simulink model "matlab_ros_com_formation1"  (R2017b)
settings: Solver=VariableStepAuto  StartTime=0.0  StopTime=inf  FixedStep=0.001  RelTol=1e-3  EnableMultiTasking=on
InitFcn:
  | sub_pose_time=0.1;
  | sub_vel_time=0.1;
  | pub_vel_time=0.1;
  | pub_pose_time=0.1;
  | 
  | Simulink.importExternalCTypes('uav.h');
undefined symbols (not defined in the file or in its folder): Pose, Twist
libraries: robotlib x28, simulink x1
settings Model: Creator=Administrator  LastModifiedBy=shitou
settings OptimizationCC: LifeSpan=inf
settings DebuggingCC: SFUnexpectedBacktrackingDiag=warning  SFNoUnconditionalDefaultTransitionDiag=warning  SFExecutionAtInitializationDiag=none
settings SFSimCC: SimCustomHeaderCode=#include <uav.h>
settings CodeAppCC: StateflowObjectComments=on
settings GRTTargetCC: TargetLangStandard=C89/C90 (ANSI)  GeneratePreprocessorConditionals=Disable all
settings ConfigComp: CovMetricSettings=dw  CovHtmlReporting=on  CovSaveCumulativeToWorkspaceVar=on  CovSaveSingleToWorkspaceVar=on  CovExternalEMLEnable=off

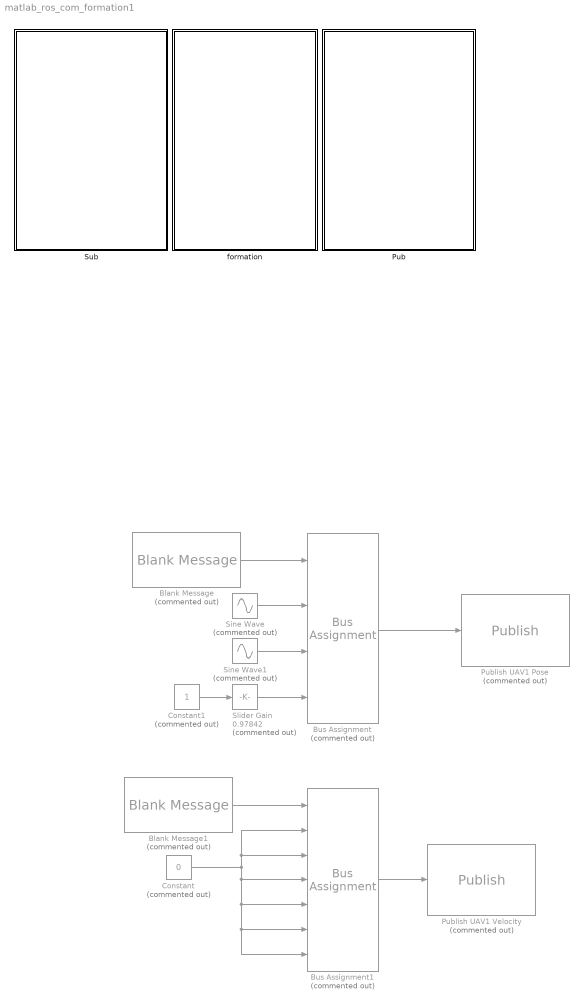
== system matlab_ros_com_formation1 ==
  Blank Message : robotlib/Blank Message  Commented=on  SourceLibraryInfo=This block requires Robotics System Toolbox  messageType=geometry_msgs/PoseStamped  SampleTime=-1
      settings: SourceProductBaseCode=RO
  Blank Message1 : robotlib/Blank Message  Commented=on  SourceLibraryInfo=This block requires Robotics System Toolbox  messageType=geometry_msgs/TwistStamped  SampleTime=inf
      settings: SourceProductBaseCode=RO
  Bus Assignment : BusAssignment  Commented=on  AssignedSignals=Pose.Position.X,Pose.Position.Y,Pose.Position.Z
  Bus Assignment1 : BusAssignment  Commented=on  AssignedSignals=Twist.Linear.X,Twist.Linear.Y,Twist.Linear.Z,Twist.Angular.X,Twist.Angular.Y,Twist.Angular.Z
  Constant : Constant  Commented=on  Value=0
  Constant1 : Constant  Commented=on
  Pub : Subsystem
  Publish UAV1 Pose : robotlib/Publish  Commented=on  SourceLibraryInfo=This block requires Robotics System Toolbox  topicSource=Specify your own  topic=uav1_matlab/mavros/local_position/pose  messageType=geometry_msgs/PoseStamped  messageQueueLength=1
      settings: SourceProductBaseCode=RO
  Publish UAV1 Velocity : robotlib/Publish  Commented=on  SourceLibraryInfo=This block requires Robotics System Toolbox  topicSource=Specify your own  topic=uav1_matlab/mavros/local_position/velocity_local  messageType=geometry_msgs/TwistStamped  messageQueueLength=1
      settings: SourceProductBaseCode=RO
  Sine Wave : Sin  Commented=on  Frequency=0.05*pi
  Sine Wave1 : Sin  Commented=on  Frequency=0.05*pi  Phase=pi/2
  Slider Gain : simulink/Math Operations/Slider Gain  Commented=on  gain=0.97842  low=0  high=2
  Sub : Subsystem
  formation : Subsystem
  wires:
  Blank Message/1 -> Bus Assignment/1
  Bus Assignment/1 -> Publish UAV1 Pose/1
  Blank Message1/1 -> Bus Assignment1/1
  Bus Assignment1/1 -> Publish UAV1 Velocity/1
  Constant1/1 -> Slider Gain/1
  Slider Gain/1 -> Bus Assignment/4
  Sine Wave/1 -> Bus Assignment/2
  Sine Wave1/1 -> Bus Assignment/3
  Constant/1 -> Bus Assignment1/7, Bus Assignment1/6, Bus Assignment1/5, Bus Assignment1/4, Bus Assignment1/3, Bus Assignment1/2

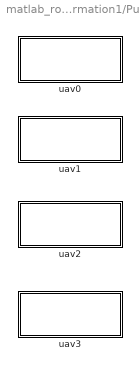
== system matlab_ros_com_formation1/Pub ==
  uav0 : Subsystem
  uav1 : Subsystem
  uav2 : Subsystem
  uav3 : Subsystem

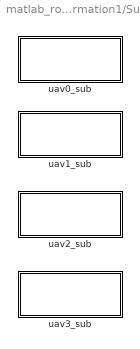
== system matlab_ros_com_formation1/Sub ==
  uav0_sub : Subsystem
  uav1_sub : Subsystem
  uav2_sub : Subsystem
  uav3_sub : Subsystem

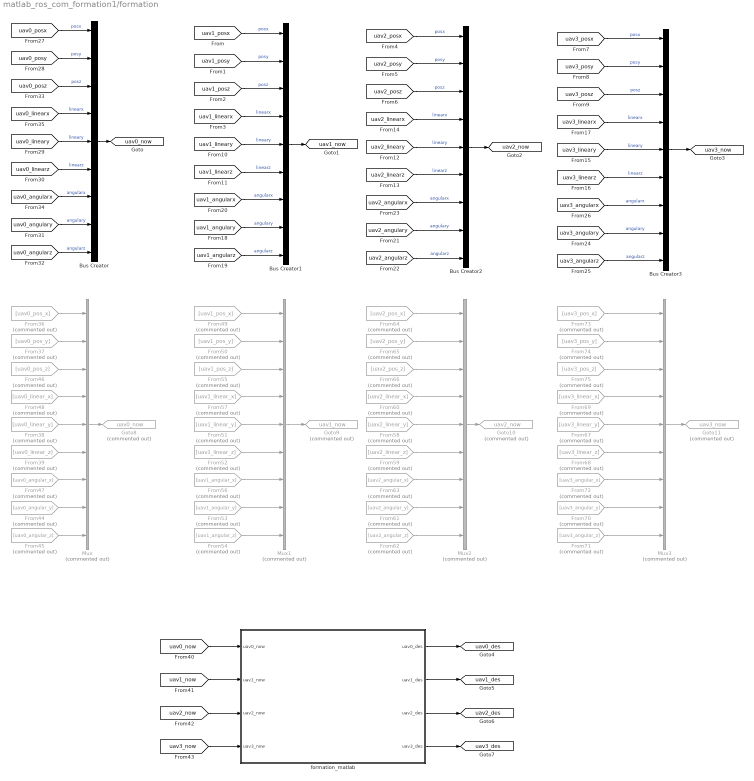
== system matlab_ros_com_formation1/formation ==
  Bus Creator{,1..3} (4 alike) : BusCreator  Inputs=9  OutDataTypeStr=Bus: uav
  From36 : From  Commented=on  GotoTag=uav0_pos_x  TagVisibility=global
  From37 : From  Commented=on  GotoTag=uav0_pos_y  TagVisibility=global
  From38 : From  Commented=on  GotoTag=uav0_linear_y  TagVisibility=global
  From39 : From  Commented=on  GotoTag=uav0_linear_z  TagVisibility=global
  From44 : From  Commented=on  GotoTag=uav0_angular_y  TagVisibility=global
  From45 : From  Commented=on  GotoTag=uav0_angular_z  TagVisibility=global
  From46 : From  Commented=on  GotoTag=uav0_pos_z  TagVisibility=global
  From47 : From  Commented=on  GotoTag=uav0_angular_x  TagVisibility=global
  From48 : From  Commented=on  GotoTag=uav0_linear_x  TagVisibility=global
  From49 : From  Commented=on  GotoTag=uav1_pos_x  TagVisibility=global
  From50 : From  Commented=on  GotoTag=uav1_pos_y  TagVisibility=global
  From51 : From  Commented=on  GotoTag=uav1_linear_y  TagVisibility=global
  From52 : From  Commented=on  GotoTag=uav1_linear_z  TagVisibility=global
  From53 : From  Commented=on  GotoTag=uav1_angular_y  TagVisibility=global
  From54 : From  Commented=on  GotoTag=uav1_angular_z  TagVisibility=global
  From55 : From  Commented=on  GotoTag=uav1_pos_z  TagVisibility=global
  From56 : From  Commented=on  GotoTag=uav1_angular_x  TagVisibility=global
  From57 : From  Commented=on  GotoTag=uav1_linear_x  TagVisibility=global
  From58 : From  Commented=on  GotoTag=uav2_linear_y  TagVisibility=global
  From59 : From  Commented=on  GotoTag=uav2_linear_z  TagVisibility=global
  From60 : From  Commented=on  GotoTag=uav2_linear_x  TagVisibility=global
  From61 : From  Commented=on  GotoTag=uav2_angular_y  TagVisibility=global
  From62 : From  Commented=on  GotoTag=uav2_angular_z  TagVisibility=global
  From63 : From  Commented=on  GotoTag=uav2_angular_x  TagVisibility=global
  From64 : From  Commented=on  GotoTag=uav2_pos_x  TagVisibility=global
  From65 : From  Commented=on  GotoTag=uav2_pos_y  TagVisibility=global
  From66 : From  Commented=on  GotoTag=uav2_pos_z  TagVisibility=global
  From67 : From  Commented=on  GotoTag=uav3_linear_y  TagVisibility=global
  From68 : From  Commented=on  GotoTag=uav3_linear_z  TagVisibility=global
  From69 : From  Commented=on  GotoTag=uav3_linear_x  TagVisibility=global
  From70 : From  Commented=on  GotoTag=uav3_angular_y  TagVisibility=global
  From71 : From  Commented=on  GotoTag=uav3_angular_z  TagVisibility=global
  From72 : From  Commented=on  GotoTag=uav3_angular_x  TagVisibility=global
  From73 : From  Commented=on  GotoTag=uav3_pos_x  TagVisibility=global
  From74 : From  Commented=on  GotoTag=uav3_pos_y  TagVisibility=global
  From75 : From  Commented=on  GotoTag=uav3_pos_z  TagVisibility=global
  Goto10 : Goto  Commented=on  GotoTag=uav2_now  TagVisibility=global
  Goto11 : Goto  Commented=on  GotoTag=uav3_now  TagVisibility=global
  Goto8 : Goto  Commented=on  GotoTag=uav0_now  TagVisibility=global
  Goto9 : Goto  Commented=on  GotoTag=uav1_now  TagVisibility=global
  Mux{,1..3} (4 alike) : Mux  Commented=on  Inputs=9
  formation_matlab : MATLAB Function  TreatAsAtomicUnit=on
  tag scope: uav0_des=global, uav0_now=global, uav1_des=global, uav1_now=global, uav2_des=global, uav2_now=global, uav3_des=global, uav3_now=global
  wires:
  [uav0_posx] -> Bus Creator/1  "posx"
  [uav0_posy] -> Bus Creator/2  "posy"
  [uav0_posz] -> Bus Creator/3  "posz"
  [uav0_linearx] -> Bus Creator/4  "linearx"
  [uav0_lineary] -> Bus Creator/5  "lineary"
  [uav0_linearz] -> Bus Creator/6  "linearz"
  [uav0_angularx] -> Bus Creator/7  "angularx"
  [uav0_angulary] -> Bus Creator/8  "angulary"
  [uav0_angularz] -> Bus Creator/9  "angularz"
  Bus Creator/1 -> [uav0_now]
  [uav1_posx] -> Bus Creator1/1  "posx"
  [uav1_posz] -> Bus Creator1/3  "posz"
  [uav1_posy] -> Bus Creator1/2  "posy"
  [uav1_linearx] -> Bus Creator1/4  "linearx"
  [uav1_lineary] -> Bus Creator1/5  "lineary"
  [uav1_linearz] -> Bus Creator1/6  "linearz"
  [uav1_angularz] -> Bus Creator1/9  "angularz"
  [uav1_angulary] -> Bus Creator1/8  "angulary"
  [uav1_angularx] -> Bus Creator1/7  "angularx"
  [uav2_posx] -> Bus Creator2/1  "posx"
  [uav2_posy] -> Bus Creator2/2  "posy"
  [uav2_posz] -> Bus Creator2/3  "posz"
  [uav2_linearx] -> Bus Creator2/4  "linearx"
  [uav2_lineary] -> Bus Creator2/5  "lineary"
  [uav2_linearz] -> Bus Creator2/6  "linearz"
  [uav2_angularx] -> Bus Creator2/7  "angularx"
  [uav2_angulary] -> Bus Creator2/8  "angulary"
  [uav2_angularz] -> Bus Creator2/9  "angularz"
  [uav3_posx] -> Bus Creator3/1  "posx"
  [uav3_angularz] -> Bus Creator3/9  "angularz"
  [uav3_angulary] -> Bus Creator3/8  "angulary"
  [uav3_angularx] -> Bus Creator3/7  "angularx"
  [uav3_linearz] -> Bus Creator3/6  "linearz"
  [uav3_lineary] -> Bus Creator3/5  "lineary"
  [uav3_linearx] -> Bus Creator3/4  "linearx"
  [uav3_posz] -> Bus Creator3/3  "posz"
  [uav3_posy] -> Bus Creator3/2  "posy"
  Bus Creator1/1 -> [uav1_now]
  Bus Creator2/1 -> [uav2_now]
  Bus Creator3/1 -> [uav3_now]
  [uav0_now] -> formation_matlab/1(uav0_now)
  [uav1_now] -> formation_matlab/2(uav1_now)
  [uav2_now] -> formation_matlab/3(uav2_now)
  [uav3_now] -> formation_matlab/4(uav3_now)
  formation_matlab/2(uav1_des) -> [uav1_des]
  formation_matlab/3(uav2_des) -> [uav2_des]
  formation_matlab/4(uav3_des) -> [uav3_des]
  From44/1 -> Mux/8
  From47/1 -> Mux/7
  From45/1 -> Mux/9
  From39/1 -> Mux/6
  From38/1 -> Mux/5
  From46/1 -> Mux/3
  From37/1 -> Mux/2
  From36/1 -> Mux/1
  From48/1 -> Mux/4
  Mux/1 -> Goto8/1
  From57/1 -> Mux1/4
  From54/1 -> Mux1/9
  From56/1 -> Mux1/7
  From49/1 -> Mux1/1
  From50/1 -> Mux1/2
  From53/1 -> Mux1/8
  From52/1 -> Mux1/6
  From55/1 -> Mux1/3
  From51/1 -> Mux1/5
  From60/1 -> Mux2/4
  From64/1 -> Mux2/1
  From63/1 -> Mux2/7
  From65/1 -> Mux2/2
  From61/1 -> Mux2/8
  From66/1 -> Mux2/3
  From58/1 -> Mux2/5
  From59/1 -> Mux2/6
  From62/1 -> Mux2/9
  From68/1 -> Mux3/6
  From69/1 -> Mux3/4
  From75/1 -> Mux3/3
  From73/1 -> Mux3/1
  From74/1 -> Mux3/2
  From71/1 -> Mux3/9
  From67/1 -> Mux3/5
  From70/1 -> Mux3/8
  From72/1 -> Mux3/7
  Mux1/1 -> Goto9/1
  Mux2/1 -> Goto10/1
  Mux3/1 -> Goto11/1
  formation_matlab/1(uav0_des) -> [uav0_des]

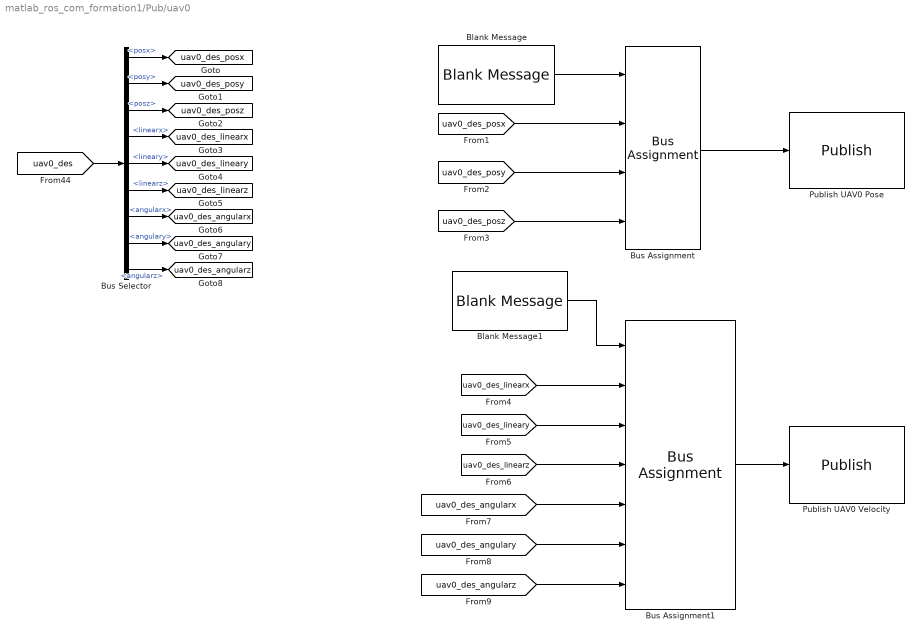
== system matlab_ros_com_formation1/Pub/uav0 ==
  Blank Message : robotlib/Blank Message  SourceLibraryInfo=This block requires Robotics System Toolbox  messageType=geometry_msgs/PoseStamped  SampleTime=pub_pose_time
      settings: SourceProductBaseCode=RO
  Blank Message1 : robotlib/Blank Message  SourceLibraryInfo=This block requires Robotics System Toolbox  messageType=geometry_msgs/TwistStamped  SampleTime=-1
      settings: SourceProductBaseCode=RO
  Bus Assignment : BusAssignment  AssignedSignals=Pose.Position.X,Pose.Position.Y,Pose.Position.Z
  Bus Assignment1 : BusAssignment  AssignedSignals=Twist.Linear.X,Twist.Linear.Y,Twist.Linear.Z,Twist.Angular.X,Twist.Angular.Y,Twist.Angular.Z
  Bus Selector : BusSelector  OutputSignals=posx,posy,posz,linearx,lineary,linearz,angularx,angulary,angularz
  Publish UAV0 Pose : robotlib/Publish  SourceLibraryInfo=This block requires Robotics System Toolbox  topicSource=Specify your own  topic=uav0_matlab/mavros/local_position/pose  messageType=geometry_msgs/PoseStamped  messageQueueLength=1
      settings: SourceProductBaseCode=RO
  Publish UAV0 Velocity : robotlib/Publish  SourceLibraryInfo=This block requires Robotics System Toolbox  topicSource=Specify your own  topic=uav0_matlab/mavros/local_position/velocity_local  messageType=geometry_msgs/TwistStamped  messageQueueLength=1
      settings: SourceProductBaseCode=RO
  tag scope: uav0_des_angularx=global, uav0_des_angulary=global, uav0_des_angularz=global, uav0_des_linearx=global, uav0_des_lineary=global, uav0_des_linearz=global, uav0_des_posx=global, uav0_des_posy=global, uav0_des_posz=global
  wires:
  Blank Message/1 -> Bus Assignment/1
  Bus Assignment/1 -> Publish UAV0 Pose/1
  Blank Message1/1 -> Bus Assignment1/1
  Bus Assignment1/1 -> Publish UAV0 Velocity/1
  [uav0_des] -> Bus Selector/1
  Bus Selector/1 -> [uav0_des_posx]  "<posx>"
  Bus Selector/3 -> [uav0_des_posz]  "<posz>"
  Bus Selector/2 -> [uav0_des_posy]  "<posy>"
  Bus Selector/4 -> [uav0_des_linearx]  "<linearx>"
  Bus Selector/5 -> [uav0_des_lineary]  "<lineary>"
  Bus Selector/6 -> [uav0_des_linearz]  "<linearz>"
  Bus Selector/7 -> [uav0_des_angularx]  "<angularx>"
  Bus Selector/8 -> [uav0_des_angulary]  "<angulary>"
  Bus Selector/9 -> [uav0_des_angularz]  "<angularz>"
  [uav0_des_posx] -> Bus Assignment/2
  [uav0_des_posy] -> Bus Assignment/3
  [uav0_des_posz] -> Bus Assignment/4
  [uav0_des_linearx] -> Bus Assignment1/2
  [uav0_des_linearz] -> Bus Assignment1/4
  [uav0_des_lineary] -> Bus Assignment1/3
  [uav0_des_angularx] -> Bus Assignment1/5
  [uav0_des_angulary] -> Bus Assignment1/6
  [uav0_des_angularz] -> Bus Assignment1/7

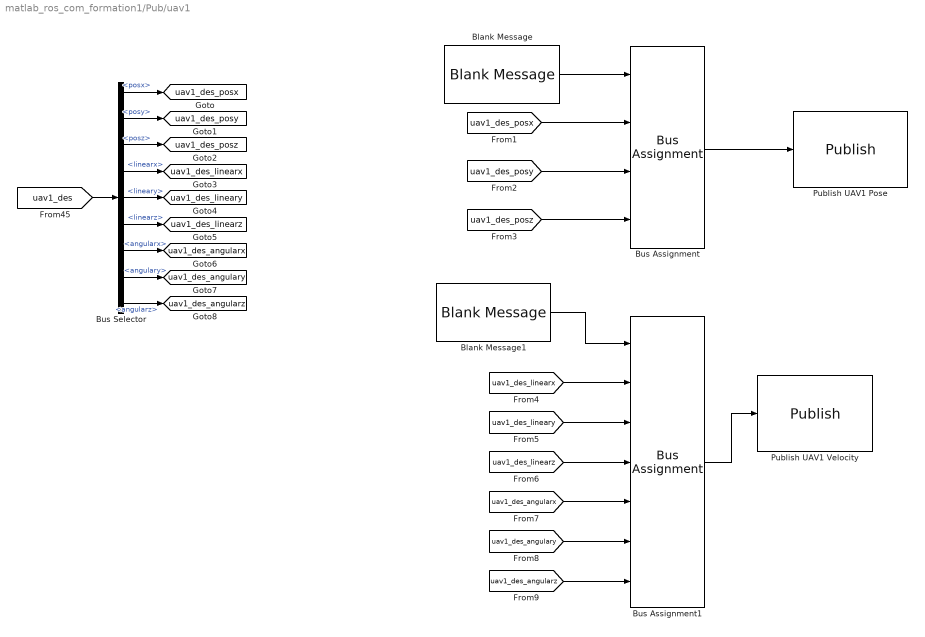
== system matlab_ros_com_formation1/Pub/uav1 ==
  Blank Message : robotlib/Blank Message  SourceLibraryInfo=This block requires Robotics System Toolbox  messageType=geometry_msgs/PoseStamped  SampleTime=pub_pose_time
      settings: SourceProductBaseCode=RO
  Blank Message1 : robotlib/Blank Message  SourceLibraryInfo=This block requires Robotics System Toolbox  messageType=geometry_msgs/TwistStamped  SampleTime=-1
      settings: SourceProductBaseCode=RO
  Bus Assignment : BusAssignment  AssignedSignals=Pose.Position.X,Pose.Position.Y,Pose.Position.Z
  Bus Assignment1 : BusAssignment  AssignedSignals=Twist.Linear.X,Twist.Linear.Y,Twist.Linear.Z,Twist.Angular.X,Twist.Angular.Y,Twist.Angular.Z
  Bus Selector : BusSelector  OutputSignals=posx,posy,posz,linearx,lineary,linearz,angularx,angulary,angularz
  Publish UAV1 Pose : robotlib/Publish  SourceLibraryInfo=This block requires Robotics System Toolbox  topicSource=Specify your own  topic=uav1_matlab/mavros/local_position/pose  messageType=geometry_msgs/PoseStamped  messageQueueLength=1
      settings: SourceProductBaseCode=RO
  Publish UAV1 Velocity : robotlib/Publish  SourceLibraryInfo=This block requires Robotics System Toolbox  topicSource=Specify your own  topic=uav1_matlab/mavros/local_position/velocity_local  messageType=geometry_msgs/TwistStamped  messageQueueLength=1
      settings: SourceProductBaseCode=RO
  tag scope: uav1_des_angularx=global, uav1_des_angulary=global, uav1_des_angularz=global, uav1_des_linearx=global, uav1_des_lineary=global, uav1_des_linearz=global, uav1_des_posx=global, uav1_des_posy=global, uav1_des_posz=global
  wires:
  Blank Message/1 -> Bus Assignment/1
  Bus Assignment/1 -> Publish UAV1 Pose/1
  Blank Message1/1 -> Bus Assignment1/1
  Bus Assignment1/1 -> Publish UAV1 Velocity/1
  [uav1_des_posz] -> Bus Assignment/4
  [uav1_des_posx] -> Bus Assignment/2
  [uav1_des_posy] -> Bus Assignment/3
  Bus Selector/2 -> [uav1_des_posy]  "<posy>"
  Bus Selector/8 -> [uav1_des_angulary]  "<angulary>"
  Bus Selector/9 -> [uav1_des_angularz]  "<angularz>"
  Bus Selector/6 -> [uav1_des_linearz]  "<linearz>"
  Bus Selector/5 -> [uav1_des_lineary]  "<lineary>"
  Bus Selector/7 -> [uav1_des_angularx]  "<angularx>"
  Bus Selector/4 -> [uav1_des_linearx]  "<linearx>"
  Bus Selector/3 -> [uav1_des_posz]  "<posz>"
  Bus Selector/1 -> [uav1_des_posx]  "<posx>"
  [uav1_des] -> Bus Selector/1
  [uav1_des_linearx] -> Bus Assignment1/2
  [uav1_des_lineary] -> Bus Assignment1/3
  [uav1_des_linearz] -> Bus Assignment1/4
  [uav1_des_angularx] -> Bus Assignment1/5
  [uav1_des_angulary] -> Bus Assignment1/6
  [uav1_des_angularz] -> Bus Assignment1/7

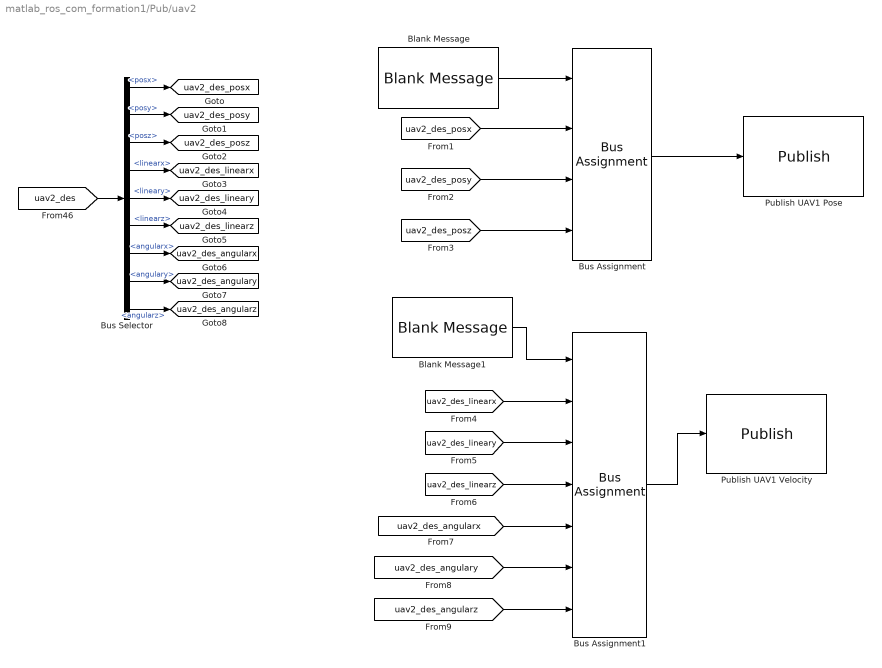
== system matlab_ros_com_formation1/Pub/uav2 ==
  Blank Message : robotlib/Blank Message  SourceLibraryInfo=This block requires Robotics System Toolbox  messageType=geometry_msgs/PoseStamped  SampleTime=pub_pose_time
      settings: SourceProductBaseCode=RO
  Blank Message1 : robotlib/Blank Message  SourceLibraryInfo=This block requires Robotics System Toolbox  messageType=geometry_msgs/TwistStamped  SampleTime=pub_vel_time
      settings: SourceProductBaseCode=RO
  Bus Assignment : BusAssignment  AssignedSignals=Pose.Position.X,Pose.Position.Y,Pose.Position.Z
  Bus Assignment1 : BusAssignment  AssignedSignals=Twist.Linear.X,Twist.Linear.Y,Twist.Linear.Z,Twist.Angular.X,Twist.Angular.Y,Twist.Angular.Z
  Bus Selector : BusSelector  OutputSignals=posx,posy,posz,linearx,lineary,linearz,angularx,angulary,angularz
  Publish UAV1 Pose : robotlib/Publish  SourceLibraryInfo=This block requires Robotics System Toolbox  topicSource=Specify your own  topic=uav2_matlab/mavros/local_position/pose  messageType=geometry_msgs/PoseStamped  messageQueueLength=1
      settings: SourceProductBaseCode=RO
  Publish UAV1 Velocity : robotlib/Publish  SourceLibraryInfo=This block requires Robotics System Toolbox  topicSource=Specify your own  topic=uav2_matlab/mavros/local_position/velocity_local  messageType=geometry_msgs/TwistStamped  messageQueueLength=1
      settings: SourceProductBaseCode=RO
  tag scope: uav2_des_angularx=global, uav2_des_angulary=global, uav2_des_angularz=global, uav2_des_linearx=global, uav2_des_lineary=global, uav2_des_linearz=global, uav2_des_posx=global, uav2_des_posy=global, uav2_des_posz=global
  wires:
  Blank Message/1 -> Bus Assignment/1
  Bus Assignment/1 -> Publish UAV1 Pose/1
  Blank Message1/1 -> Bus Assignment1/1
  Bus Assignment1/1 -> Publish UAV1 Velocity/1
  [uav2_des_linearx] -> Bus Assignment1/2
  [uav2_des_lineary] -> Bus Assignment1/3
  [uav2_des_linearz] -> Bus Assignment1/4
  [uav2_des_angularx] -> Bus Assignment1/5
  [uav2_des_angulary] -> Bus Assignment1/6
  [uav2_des_angularz] -> Bus Assignment1/7
  [uav2_des_posx] -> Bus Assignment/2
  [uav2_des_posy] -> Bus Assignment/3
  [uav2_des_posz] -> Bus Assignment/4
  Bus Selector/1 -> [uav2_des_posx]  "<posx>"
  Bus Selector/3 -> [uav2_des_posz]  "<posz>"
  Bus Selector/4 -> [uav2_des_linearx]  "<linearx>"
  Bus Selector/6 -> [uav2_des_linearz]  "<linearz>"
  Bus Selector/5 -> [uav2_des_lineary]  "<lineary>"
  Bus Selector/8 -> [uav2_des_angulary]  "<angulary>"
  Bus Selector/2 -> [uav2_des_posy]  "<posy>"
  Bus Selector/9 -> [uav2_des_angularz]  "<angularz>"
  Bus Selector/7 -> [uav2_des_angularx]  "<angularx>"
  [uav2_des] -> Bus Selector/1

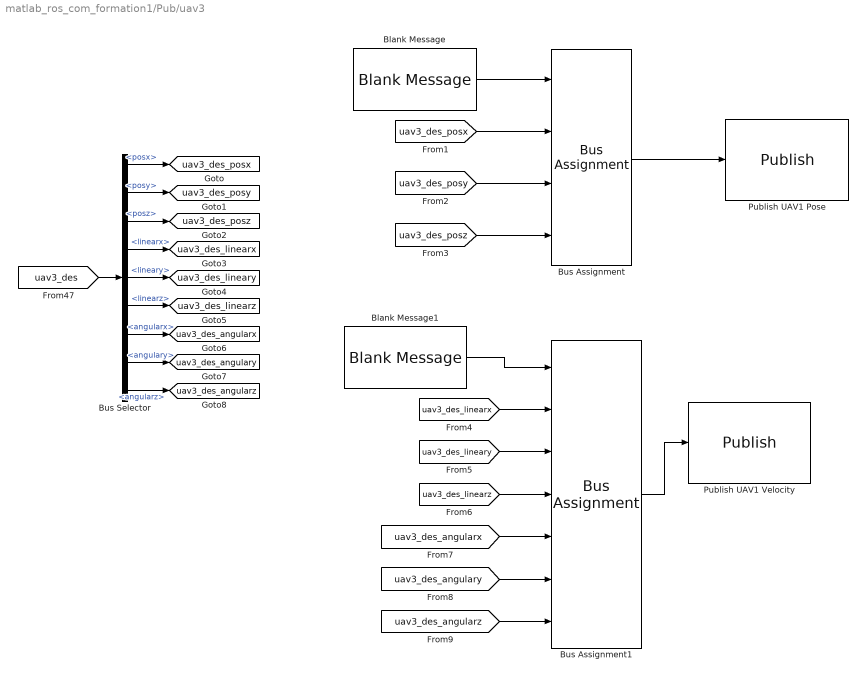
== system matlab_ros_com_formation1/Pub/uav3 ==
  Blank Message : robotlib/Blank Message  SourceLibraryInfo=This block requires Robotics System Toolbox  messageType=geometry_msgs/PoseStamped  SampleTime=pub_pose_time
      settings: SourceProductBaseCode=RO
  Blank Message1 : robotlib/Blank Message  SourceLibraryInfo=This block requires Robotics System Toolbox  messageType=geometry_msgs/TwistStamped  SampleTime=pub_vel_time
      settings: SourceProductBaseCode=RO
  Bus Assignment : BusAssignment  AssignedSignals=Pose.Position.X,Pose.Position.Y,Pose.Position.Z
  Bus Assignment1 : BusAssignment  AssignedSignals=Twist.Linear.X,Twist.Linear.Y,Twist.Linear.Z,Twist.Angular.X,Twist.Angular.Y,Twist.Angular.Z
  Bus Selector : BusSelector  OutputSignals=posx,posy,posz,linearx,lineary,linearz,angularx,angulary,angularz
  Publish UAV1 Pose : robotlib/Publish  SourceLibraryInfo=This block requires Robotics System Toolbox  topicSource=Specify your own  topic=uav3_matlab/mavros/local_position/pose  messageType=geometry_msgs/PoseStamped  messageQueueLength=1
      settings: SourceProductBaseCode=RO
  Publish UAV1 Velocity : robotlib/Publish  SourceLibraryInfo=This block requires Robotics System Toolbox  topicSource=Specify your own  topic=uav3_matlab/mavros/local_position/velocity_local  messageType=geometry_msgs/TwistStamped  messageQueueLength=1
      settings: SourceProductBaseCode=RO
  tag scope: uav3_des_angularx=global, uav3_des_angulary=global, uav3_des_angularz=global, uav3_des_linearx=global, uav3_des_lineary=global, uav3_des_linearz=global, uav3_des_posx=global, uav3_des_posy=global, uav3_des_posz=global
  wires:
  Blank Message/1 -> Bus Assignment/1
  Bus Assignment/1 -> Publish UAV1 Pose/1
  Blank Message1/1 -> Bus Assignment1/1
  Bus Assignment1/1 -> Publish UAV1 Velocity/1
  [uav3_des_posx] -> Bus Assignment/2
  [uav3_des_posy] -> Bus Assignment/3
  [uav3_des_posz] -> Bus Assignment/4
  [uav3_des_linearx] -> Bus Assignment1/2
  [uav3_des_lineary] -> Bus Assignment1/3
  [uav3_des_linearz] -> Bus Assignment1/4
  [uav3_des_angularx] -> Bus Assignment1/5
  [uav3_des_angulary] -> Bus Assignment1/6
  [uav3_des_angularz] -> Bus Assignment1/7
  Bus Selector/1 -> [uav3_des_posx]  "<posx>"
  Bus Selector/3 -> [uav3_des_posz]  "<posz>"
  Bus Selector/4 -> [uav3_des_linearx]  "<linearx>"
  Bus Selector/6 -> [uav3_des_linearz]  "<linearz>"
  Bus Selector/5 -> [uav3_des_lineary]  "<lineary>"
  Bus Selector/8 -> [uav3_des_angulary]  "<angulary>"
  Bus Selector/2 -> [uav3_des_posy]  "<posy>"
  Bus Selector/9 -> [uav3_des_angularz]  "<angularz>"
  Bus Selector/7 -> [uav3_des_angularx]  "<angularx>"
  [uav3_des] -> Bus Selector/1

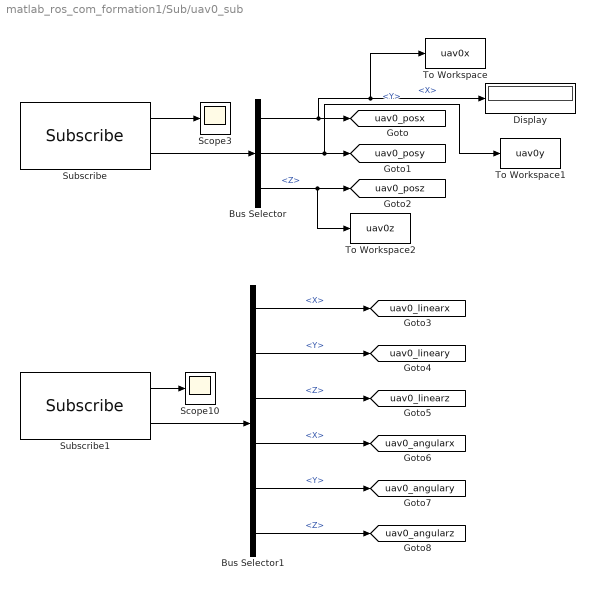
== system matlab_ros_com_formation1/Sub/uav0_sub ==
  Bus Selector : BusSelector  OutputSignals=Pose.Position.X,Pose.Position.Y,Pose.Position.Z
  Bus Selector1 : BusSelector  OutputSignals=Twist.Linear.X,Twist.Linear.Y,Twist.Linear.Z,Twist.Angular.X,Twist.Angular.Y,Twist.Angular.Z
  Display : Display
  Scope10 : Scope
  Scope3 : Scope
  Subscribe : robotlib/Subscribe  SourceLibraryInfo=This block requires Robotics System Toolbox  topicSource=Select from ROS network  topic=/uav0/mavros/local_position/pose  messageType=geometry_msgs/PoseStamped  sampleTime=sub_pose_time  messageQueueLength=1
      settings: SourceProductBaseCode=RO
  Subscribe1 : robotlib/Subscribe  SourceLibraryInfo=This block requires Robotics System Toolbox  topicSource=Select from ROS network  topic=/uav0/mavros/local_position/velocity_local  messageType=geometry_msgs/TwistStamped  sampleTime=sub_vel_time  messageQueueLength=1
      settings: SourceProductBaseCode=RO
  To Workspace : ToWorkspace  VariableName=uav0x  SaveFormat=Structure With Time  SampleTime=-1
  To Workspace1 : ToWorkspace  VariableName=uav0y  SaveFormat=Structure With Time  SampleTime=-1
  To Workspace2 : ToWorkspace  VariableName=uav0z  SaveFormat=Structure With Time  SampleTime=-1
  tag scope: uav0_angularx=global, uav0_angulary=global, uav0_angularz=global, uav0_linearx=global, uav0_lineary=global, uav0_linearz=global, uav0_posx=global, uav0_posy=global, uav0_posz=global
  wires:
  Subscribe/1 -> Scope3/1
  Subscribe/2 -> Bus Selector/1
  Bus Selector/1 -> To Workspace/1, Display/1, [uav0_posx]  "<X>"
  Bus Selector/2 -> To Workspace1/1, [uav0_posy]  "<Y>"
  Bus Selector/3 -> To Workspace2/1, [uav0_posz]  "<Z>"
  Subscribe1/2 -> Bus Selector1/1
  Subscribe1/1 -> Scope10/1
  Bus Selector1/1 -> [uav0_linearx]  "<X>"
  Bus Selector1/2 -> [uav0_lineary]  "<Y>"
  Bus Selector1/3 -> [uav0_linearz]  "<Z>"
  Bus Selector1/4 -> [uav0_angularx]  "<X>"
  Bus Selector1/5 -> [uav0_angulary]  "<Y>"
  Bus Selector1/6 -> [uav0_angularz]  "<Z>"

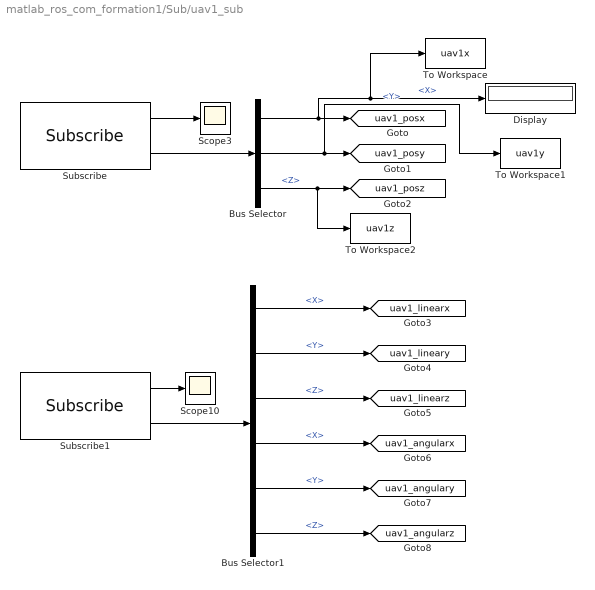
== system matlab_ros_com_formation1/Sub/uav1_sub ==
  Bus Selector : BusSelector  OutputSignals=Pose.Position.X,Pose.Position.Y,Pose.Position.Z
  Bus Selector1 : BusSelector  OutputSignals=Twist.Linear.X,Twist.Linear.Y,Twist.Linear.Z,Twist.Angular.X,Twist.Angular.Y,Twist.Angular.Z
  Display : Display
  Scope10 : Scope
  Scope3 : Scope
  Subscribe : robotlib/Subscribe  SourceLibraryInfo=This block requires Robotics System Toolbox  topicSource=Select from ROS network  topic=/uav1/mavros/local_position/pose  messageType=geometry_msgs/PoseStamped  sampleTime=sub_pose_time  messageQueueLength=1
      settings: SourceProductBaseCode=RO
  Subscribe1 : robotlib/Subscribe  SourceLibraryInfo=This block requires Robotics System Toolbox  topicSource=Select from ROS network  topic=/uav1/mavros/local_position/velocity_local  messageType=geometry_msgs/TwistStamped  sampleTime=sub_vel_time  messageQueueLength=1
      settings: SourceProductBaseCode=RO
  To Workspace : ToWorkspace  VariableName=uav1x  SaveFormat=Structure With Time  SampleTime=-1
  To Workspace1 : ToWorkspace  VariableName=uav1y  SaveFormat=Structure With Time  SampleTime=-1
  To Workspace2 : ToWorkspace  VariableName=uav1z  SaveFormat=Structure With Time  SampleTime=-1
  tag scope: uav1_angularx=global, uav1_angulary=global, uav1_angularz=global, uav1_linearx=global, uav1_lineary=global, uav1_linearz=global, uav1_posx=global, uav1_posy=global, uav1_posz=global
  wires:
  Subscribe/1 -> Scope3/1
  Subscribe/2 -> Bus Selector/1
  Bus Selector/1 -> To Workspace/1, Display/1, [uav1_posx]  "<X>"
  Bus Selector/2 -> To Workspace1/1, [uav1_posy]  "<Y>"
  Bus Selector/3 -> To Workspace2/1, [uav1_posz]  "<Z>"
  Subscribe1/2 -> Bus Selector1/1
  Subscribe1/1 -> Scope10/1
  Bus Selector1/1 -> [uav1_linearx]  "<X>"
  Bus Selector1/2 -> [uav1_lineary]  "<Y>"
  Bus Selector1/3 -> [uav1_linearz]  "<Z>"
  Bus Selector1/4 -> [uav1_angularx]  "<X>"
  Bus Selector1/5 -> [uav1_angulary]  "<Y>"
  Bus Selector1/6 -> [uav1_angularz]  "<Z>"

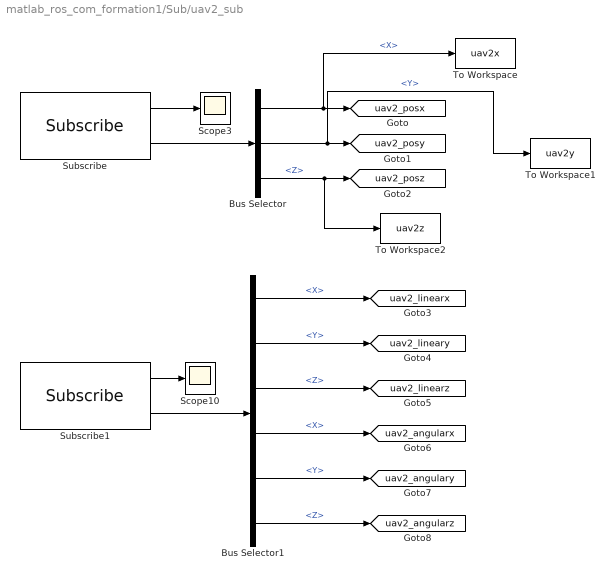
== system matlab_ros_com_formation1/Sub/uav2_sub ==
  Bus Selector : BusSelector  OutputSignals=Pose.Position.X,Pose.Position.Y,Pose.Position.Z
  Bus Selector1 : BusSelector  OutputSignals=Twist.Linear.X,Twist.Linear.Y,Twist.Linear.Z,Twist.Angular.X,Twist.Angular.Y,Twist.Angular.Z
  Scope10 : Scope
  Scope3 : Scope
  Subscribe : robotlib/Subscribe  SourceLibraryInfo=This block requires Robotics System Toolbox  topicSource=Select from ROS network  topic=/uav2/mavros/local_position/pose  messageType=geometry_msgs/PoseStamped  sampleTime=sub_pose_time  messageQueueLength=1
      settings: SourceProductBaseCode=RO
  Subscribe1 : robotlib/Subscribe  SourceLibraryInfo=This block requires Robotics System Toolbox  topicSource=Select from ROS network  topic=/uav2/mavros/local_position/velocity_local  messageType=geometry_msgs/TwistStamped  sampleTime=sub_vel_time  messageQueueLength=1
      settings: SourceProductBaseCode=RO
  To Workspace : ToWorkspace  VariableName=uav2x  SaveFormat=Structure With Time  SampleTime=-1
  To Workspace1 : ToWorkspace  VariableName=uav2y  SaveFormat=Structure With Time  SampleTime=-1
  To Workspace2 : ToWorkspace  VariableName=uav2z  SaveFormat=Structure With Time  SampleTime=-1
  tag scope: uav2_angularx=global, uav2_angulary=global, uav2_angularz=global, uav2_linearx=global, uav2_lineary=global, uav2_linearz=global, uav2_posx=global, uav2_posy=global, uav2_posz=global
  wires:
  Subscribe/1 -> Scope3/1
  Subscribe/2 -> Bus Selector/1
  Bus Selector/1 -> To Workspace/1, [uav2_posx]  "<X>"
  Bus Selector/2 -> To Workspace1/1, [uav2_posy]  "<Y>"
  Bus Selector/3 -> To Workspace2/1, [uav2_posz]  "<Z>"
  Subscribe1/2 -> Bus Selector1/1
  Subscribe1/1 -> Scope10/1
  Bus Selector1/1 -> [uav2_linearx]  "<X>"
  Bus Selector1/2 -> [uav2_lineary]  "<Y>"
  Bus Selector1/3 -> [uav2_linearz]  "<Z>"
  Bus Selector1/4 -> [uav2_angularx]  "<X>"
  Bus Selector1/5 -> [uav2_angulary]  "<Y>"
  Bus Selector1/6 -> [uav2_angularz]  "<Z>"

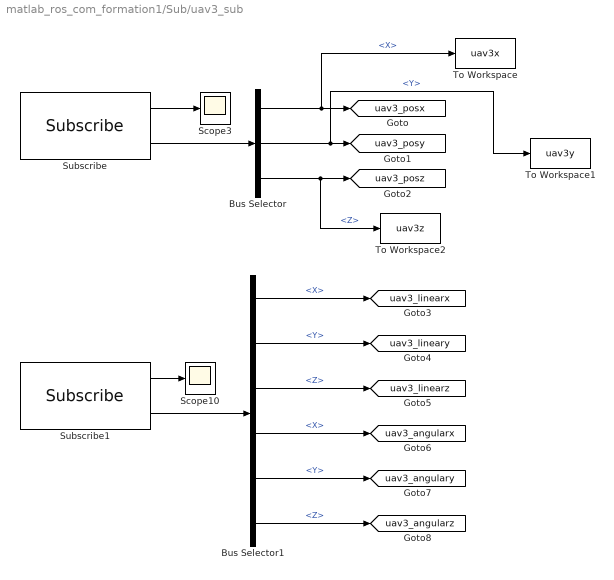
== system matlab_ros_com_formation1/Sub/uav3_sub ==
  Bus Selector : BusSelector  OutputSignals=Pose.Position.X,Pose.Position.Y,Pose.Position.Z
  Bus Selector1 : BusSelector  OutputSignals=Twist.Linear.X,Twist.Linear.Y,Twist.Linear.Z,Twist.Angular.X,Twist.Angular.Y,Twist.Angular.Z
  Scope10 : Scope
  Scope3 : Scope
  Subscribe : robotlib/Subscribe  SourceLibraryInfo=This block requires Robotics System Toolbox  topicSource=Select from ROS network  topic=/uav3/mavros/local_position/pose  messageType=geometry_msgs/PoseStamped  sampleTime=sub_pose_time  messageQueueLength=1
      settings: SourceProductBaseCode=RO
  Subscribe1 : robotlib/Subscribe  SourceLibraryInfo=This block requires Robotics System Toolbox  topicSource=Select from ROS network  topic=/uav3/mavros/local_position/velocity_local  messageType=geometry_msgs/TwistStamped  sampleTime=sub_vel_time  messageQueueLength=1
      settings: SourceProductBaseCode=RO
  To Workspace : ToWorkspace  VariableName=uav3x  SaveFormat=Structure With Time  SampleTime=-1
  To Workspace1 : ToWorkspace  VariableName=uav3y  SaveFormat=Structure With Time  SampleTime=-1
  To Workspace2 : ToWorkspace  VariableName=uav3z  SaveFormat=Structure With Time  SampleTime=-1
  tag scope: uav3_angularx=global, uav3_angulary=global, uav3_angularz=global, uav3_linearx=global, uav3_lineary=global, uav3_linearz=global, uav3_posx=global, uav3_posy=global, uav3_posz=global
  wires:
  Subscribe/1 -> Scope3/1
  Subscribe/2 -> Bus Selector/1
  Bus Selector/1 -> To Workspace/1, [uav3_posx]  "<X>"
  Bus Selector/2 -> To Workspace1/1, [uav3_posy]  "<Y>"
  Bus Selector/3 -> To Workspace2/1, [uav3_posz]  "<Z>"
  Subscribe1/2 -> Bus Selector1/1
  Subscribe1/1 -> Scope10/1
  Bus Selector1/1 -> [uav3_linearx]  "<X>"
  Bus Selector1/2 -> [uav3_lineary]  "<Y>"
  Bus Selector1/3 -> [uav3_linearz]  "<Z>"
  Bus Selector1/4 -> [uav3_angularx]  "<X>"
  Bus Selector1/5 -> [uav3_angulary]  "<Y>"
  Bus Selector1/6 -> [uav3_angularz]  "<Z>"

== matlab function matlab_ros_com_formation1/formation/formation_matlab ==
  data: uav0_now input Bus: uav; uav0_des output Bus: uav; uav1_now input Bus: uav; uav2_now input Bus: uav; uav3_now input Bus: uav; uav1_des output Bus: uav; uav2_des output Bus: uav; uav3_des output Bus: uav
function [uav0_des,uav1_des,uav2_des,uav3_des ] = formation_matlab(uav0_now,uav1_now,uav2_now,uav3_now)

% formation.Ppos_now=[uav0.now,uav1.now,uav2.now,uav3.now];
%%%%%%虚拟领导者位置
leader.posx=0;
leader.posy=0;
leader.posz=0;
T_SIZE=2.0;
k_aij=0.1;
% k_p=0.95;
k_p=1.95;


relative_pos_to_leader0.x = -T_SIZE;
relative_pos_to_leader0.y =  T_SIZE;
relative_pos_to_leader0.z = 0.0;

relative_pos_to_leader1.x =   T_SIZE;
relative_pos_to_leader1.y =   T_SIZE;
relative_pos_to_leader1.z = 0.0;
    
relative_pos_to_leader2.x =   T_SIZE;
relative_pos_to_leader2.y = - T_SIZE;
relative_pos_to_leader2.z = 0.0;
   
relative_pos_to_leader3.x = - T_SIZE;
relative_pos_to_leader3.y = - T_SIZE;
relative_pos_to_leader3.z = 0.0;
   


uav0_des.posx = 0;
uav0_des.posy = 0;
uav0_des.posz = 1.0;    
uav0_des.linearx = k_p * (leader.posx + relative_pos_to_leader0.x - uav0_now.posx) + k_aij*( uav1_now.posx - uav0_now.posx) + k_aij*( uav3_now.posx - uav0_now.posx);
uav0_des.lineary = k_p * (leader.posy + relative_pos_to_leader0.y - uav0_now.posy) + k_aij*( uav1_now.posy - uav0_now.posy) + k_aij*( uav3_now.posy - uav0_now.posy);
uav0_des.linearz = 0;
uav0_des.angularx = 0;
uav0_des.angulary = 0;
uav0_des.angularz = 0;

uav1_des.posx = 0;
uav1_des.posy = 0;
uav1_des.posz = 2.0;
uav1_des.linearx = k_p * (leader.posx + relative_pos_to_leader1.x - uav1_now.posx) + k_aij*( uav0_now.posx - uav1_now.posx) + k_aij*( uav2_now.posx - uav1_now.posx);
uav1_des.lineary = k_p * (leader.posy + relative_pos_to_leader1.y - uav1_now.posy) + k_aij*( uav0_now.posy - uav1_now.posy) + k_aij*( uav2_now.posy - uav1_now.posy);
uav1_des.linearz = 0;
uav1_des.angularx = 0;
uav1_des.angulary = 0;
uav1_des.angularz = 0;

uav2_des.posx = 0;
uav2_des.posy = 0;
uav2_des.posz = 3.0;
uav2_des.linearx = k_p * (leader.posx + relative_pos_to_leader2.x - uav2_now.posx) + k_aij*( uav1_now.posx - uav2_now.posx) + k_aij*( uav3_now.posx - uav2_now.posx);
uav2_des.lineary = k_p * (leader.posy + relative_pos_to_leader2.y - uav2_now.posy) + k_aij*( uav1_now.posy - uav2_now.posy) + k_aij*( uav3_now.posy - uav2_now.posy);
uav2_des.linearz = 0;
uav2_des.angularx = 0;
uav2_des.angulary = 0;
uav2_des.angularz = 0;

uav3_des.posx = 0;
uav3_des.posy = 0;
uav3_des.posz = 4.0;
uav3_des.linearx = k_p * (leader.posx + relative_pos_to_leader3.x - uav3_now.posx) + k_aij*( uav0_now.posx - uav3_now.posx) + k_aij*( uav2_now.posx - uav3_now.posx);
uav3_des.lineary = k_p * (leader.posy + relative_pos_to_leader3.y - uav3_now.posy) + k_aij*( uav0_now.posy - uav3_now.posy) + k_aij*( uav2_now.posy - uav3_now.posy);
uav3_des.linearz = 0;
uav3_des.angularx = 0;
uav3_des.angulary = 0;
uav3_des.angularz = 0;
end
